simulink model "Project_Model_simulink_version_12_7_2023"  (R2021a)
settings: Solver=FixedStepDiscrete  StartTime=0.0  StopTime=10  FixedStep=0.2  RelTol=1e-3
values from neighbouring files (symbols this model uses):
  C = 120    [project_script.m]
  Hp = 160    [project_script.m]
  Im1 = 180    [project_script.m]
  Im2 = 315    [project_script.m]
  Im3 = 225    [project_script.m]
  Im4 = 270    [project_script.m]
  Ip1 = 177.5    [project_script.m]
  Ip2 = 312.5    [project_script.m]
  Ip3 = 222.5    [project_script.m]
  Ip4 = 267.5    [project_script.m]
  Lp = 10    [project_script.m]
  RPMC = 6000    [project_script.m]
  Tcr = 1/360    (= 0.00277777777778)    [project_script.m]
  Tinc = 1.05    [project_script.m]
  Tmax = 90    [project_script.m]
  Tmi = 4.5/360    (= 0.0125)    [project_script.m]
  Tpi = 2/360    (= 0.00555555555556)    [project_script.m]
undefined symbols (not defined in the file or in its folder): sigbuilder_block
(part 2 of 2)

== system Project_Model_simulink_version_12_7_2023/CRDI_Integrated_Fuel_Injection_system/Injector_Subsystem/Injector4/Injector_2Subsystem/Main_injection ==
  Crank_angle : Inport  OutDataTypeStr=single
  Total_ontime_maininjection : Inport  Port=2  OutDataTypeStr=single
  Time_for_1_Degree : Inport  Port=3  OutDataTypeStr=single
  Add : Sum  AccumDataTypeStr=single
      settings: AttributesFormatString=AccumDataTypeStr=%<AccumDataTypeStr>
  Divide : Product  Inputs=*/  OutDataTypeStr=single
  Logical Operator : Logic  AllPortsSameDT=off  OutDataTypeStr=boolean
  Main_Inj_trg_angle_inj1 : Constant  Value=Im4
  Main_Inj_trg_angle_inj2 : Constant  Value=Im4
  Relational Operator : RelationalOperator  OutDataTypeStr=boolean  RndMeth=Simplest
  Relational Operator1 : RelationalOperator  Operator=<=  OutDataTypeStr=boolean  RndMeth=Simplest
  main_inj_on_off_signal : Outport  VectorParamsAs1DForOutWhenUnconnected=off
  wires:
  Logical Operator/1 -> main_inj_on_off_signal/1  "main_inj_on_off_signal"
  Time_for_1_Degree/1 -> Divide/2
  Relational Operator/1 -> Logical Operator/1
  Main_Inj_trg_angle_inj2/1 -> Add/1
  Add/1 -> Relational Operator1/2  "Total_On_Degree"
  Crank_angle/1 -> Relational Operator1/1, Relational Operator/1
  Main_Inj_trg_angle_inj1/1 -> Relational Operator/2
  Relational Operator1/1 -> Logical Operator/2
  Total_ontime_maininjection/1 -> Divide/1
  Divide/1 -> Add/2

== system Project_Model_simulink_version_12_7_2023/CRDI_Integrated_Fuel_Injection_system/Injector_Subsystem/Injector4/Injector_2Subsystem/Pre_injection ==
  Crank_angle : Inport  OutDataTypeStr=single
  Total_ontime_preinjection : Inport  Port=2  OutDataTypeStr=single
  Time_For_1_Degree : Inport  Port=3  OutDataTypeStr=single
  Add : Sum  AccumDataTypeStr=single
      settings: AttributesFormatString=AccumDataTypeStr=%<AccumDataTypeStr>
  Divide : Product  Inputs=*/  OutDataTypeStr=single
  Logical Operator : Logic  AllPortsSameDT=off  OutDataTypeStr=boolean
  Pre_Inj_trg_angle_inj1 : Constant  Value=Ip4
  Pre_Inj_trg_angle_inj2 : Constant  Value=Ip4
  Relational Operator : RelationalOperator  OutDataTypeStr=boolean  RndMeth=Simplest
  Relational Operator1 : RelationalOperator  Operator=<=  OutDataTypeStr=boolean  RndMeth=Simplest
  pre_inj_on_off_signal : Outport  VectorParamsAs1DForOutWhenUnconnected=off
  wires:
  Divide/1 -> Add/2
  Relational Operator1/1 -> Logical Operator/2
  Pre_Inj_trg_angle_inj1/1 -> Relational Operator/2  "<Trigger_angle>"
  Total_ontime_preinjection/1 -> Divide/1
  Add/1 -> Relational Operator1/2  "Total_On_Degree"
  Pre_Inj_trg_angle_inj2/1 -> Add/1  "<Trigger_angle>"
  Time_For_1_Degree/1 -> Divide/2
  Relational Operator/1 -> Logical Operator/1
  Crank_angle/1 -> Relational Operator1/1, Relational Operator/1
  Logical Operator/1 -> pre_inj_on_off_signal/1  "pre_inj_on_off_signal"

== system Project_Model_simulink_version_12_7_2023/CRDI_Integrated_Fuel_Injection_system/Injector_Subsystem/Injector4/Injector_2Subsystem/Subsystem ==
  note: Subsystem
      | Description: Integrates Pre, Main, Post Injection to single output
      | Input: On time for pre Injection, On time for main Injection, On time for post Injection, Pre Pulse, Main Pulse, Post Pulse
      | Output: On time for Injection
  On_Time_Pre_Injection : Inport
  Pre_Pulse : Inport  Port=2
  On_Time_Main_Injection : Inport  Port=3
  Main_Pulse : Inport  Port=4
  Constant : Constant  Value=0
  Switch1 : Switch  Criteria=u2 ~= 0
  Switch2 : Switch  Criteria=u2 ~= 0
  Enable_Disable : Outport  VectorParamsAs1DForOutWhenUnconnected=off
  wires:
  Main_Pulse/1 -> Switch2/2
  On_Time_Main_Injection/1 -> Switch2/1
  Pre_Pulse/1 -> Switch1/2
  On_Time_Pre_Injection/1 -> Switch1/1
  Switch1/1 -> Enable_Disable/1  "On_Time_Injection"
  Constant/1 -> Switch2/3  "constant"
  Switch2/1 -> Switch1/3

== matlab function Project_Model_simulink_version_12_7_2023/CRDI_Integrated_Fuel_Injection_system/Sensors_Subsystem/Oxygen sensor/MATLAB Function ==
  data: u input; out output
function out = fcn(u)
%#codegen

if (u>0.65)
y = 0.95;
elseif (u<=0.65 && u>=0.25)
    y = 1;
else
    y=1.05;
end

out=y;
